simulink model "sim_sys_scara"  (R2017a)
settings: Solver=VariableStepAuto  StartTime=0.0  StopTime=4.1  MaxStep=0.01  RelTol=1e-4  EnableMultiTasking=on
values from neighbouring files (symbols this model uses):
  n_juncoes = size(vars, 1)    [animation.m]    (also in puma.m = 4; scara.m = 4)
undefined symbols (not defined in the file or in its folder): Q0
libraries: simulink x1
settings Model: Creator=julio  LastModifiedBy=julio
settings DataIOCC: LimitDataPoints=on  SaveOutput=off  SaveTime=off
settings OptimizationCC: ExpressionDepthLimit=2147483647  LifeSpan=1
settings DebuggingCC: AlgebraicLoopMsg=none  UnderspecifiedInitializationDetection=Classic  MergeDetectMultiDrivingBlocksExec=none  FcnCallInpInsideContextMsg=warning  AllowSymbolicDim=off  StateNameClashWarn=warning  SFUnexpectedBacktrackingDiag=warning  SFNoUnconditionalDefaultTransitionDiag=warning  SFExecutionAtInitializationDiag=none
settings GRTTargetCC: TargetLangStandard=C89/C90 (ANSI)  GeneratePreprocessorConditionals=Disable all  CombineOutputUpdateFcns=off  GRTInterface=on

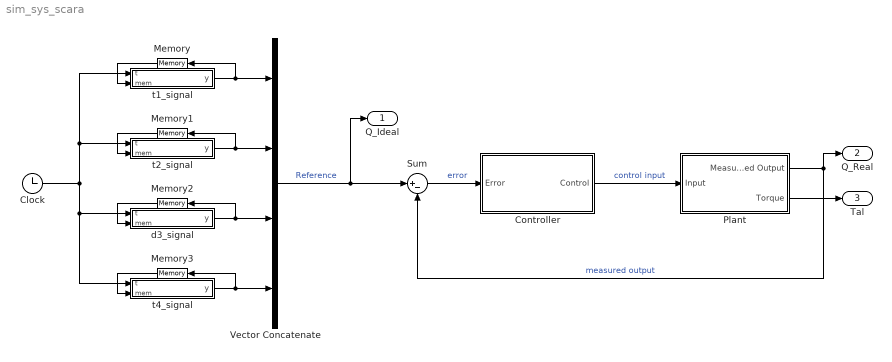
== system sim_sys_scara ==
  Clock : Clock
  Controller : Subsystem
  Memory : Memory  X0=Q0(1)
  Memory1 : Memory  X0=Q0(2)
  Memory2 : Memory  X0=Q0(3)
  Memory3 : Memory  X0=Q0(4)
  Plant : Subsystem
  Sum : Sum  Inputs=|+-
  Vector Concatenate : Concatenate  NumInputs=4
  d3_signal : MATLAB Function  TreatAsAtomicUnit=on
  t1_signal : MATLAB Function  TreatAsAtomicUnit=on
  t2_signal : MATLAB Function  TreatAsAtomicUnit=on
  t4_signal : MATLAB Function  TreatAsAtomicUnit=on
  Q_Ideal : Outport
  Q_Real : Outport  Port=2
  Tal : Outport  Port=3
  wires:
  Plant/1(Measured Output) -> Sum/2, Q_Real/1  "measured output"
  Sum/1 -> Controller/1(Error)  "error"
  Controller/1(Control) -> Plant/1(Input)  "control input"
  Vector Concatenate/1 -> Q_Ideal/1, Sum/1  "Reference"
  t1_signal/1(y) -> Memory/1, Vector Concatenate/1
  Memory/1 -> t1_signal/2(mem)
  Memory1/1 -> t2_signal/2(mem)
  t2_signal/1(y) -> Vector Concatenate/2, Memory1/1
  Memory2/1 -> d3_signal/2(mem)
  d3_signal/1(y) -> Vector Concatenate/3, Memory2/1
  Memory3/1 -> t4_signal/2(mem)
  t4_signal/1(y) -> Vector Concatenate/4, Memory3/1
  Clock/1 -> d3_signal/1(t), t4_signal/1(t), t2_signal/1(t), t1_signal/1(t)
  Plant/2(Torque) -> Tal/1

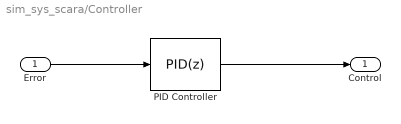
== system sim_sys_scara/Controller ==
  Error : Inport  PortDimensions=n_juncoes
  PID Controller : simulink/Continuous/PID Controller  Controller=PID  TimeDomain=Discrete-time  SampleTime=0.01  IntegratorMethod=Forward Euler  FilterMethod=Forward Euler  Form=Ideal  UseFilter=off  ControllerParametersSource=internal  P=8  I=5  D=10  N=20  InitialConditionSource=internal  InitialConditionForIntegrator=0  InitialConditionForFilter=0  ExternalReset=none  LimitOutput=off  UpperSaturationLimit=inf  LowerSaturationLimit=-inf  LinearizeAsGain=on  AntiWindupMode=none  Kb=1  TrackingMode=off  Kt=1  PParamMin=[]  PParamMax=[]  IParamMin=[]  IParamMax=[]  DParamMin=[]  DParamMax=[]  NParamMin=[]  NParamMax=[]  KbParamMin=[]  KbParamMax=[]  KtParamMin=[]  KtParamMax=[]  POutMin=[]  POutMax=[]  IOutMin=[]  IOutMax=[]  DOutMin=[]  DOutMax=[]  NOutMin=[]  NOutMax=[]  KbOutMin=[]  KbOutMax=[]  KtOutMin=[]  KtOutMax=[]  IntegratorOutMin=[]  IntegratorOutMax=[]  FilterOutMin=[]  FilterOutMax=[]  SumOutMin=[]  SumOutMax=[]  SumI1OutMin=[]  SumI1OutMax=[]  SumI2OutMin=[]  SumI2OutMax=[]  SumI3OutMin=[]  SumI3OutMax=[]  SumDOutMin=[]  SumDOutMax=[]  SaturationOutMin=[]  SaturationOutMax=[]  IntegratorContinuousStateAttributes=''  IntegratorStateMustResolveToSignalObject=off  IntegratorRTWStateStorageClass=Auto  FilterContinuousStateAttributes=''  FilterStateMustResolveToSignalObject=off  FilterRTWStateStorageClass=Auto  DifferentiatorICPrevScaledInput=0  DifferentiatorOutMin=[]  DifferentiatorOutMax=[]  InitialConditionSetting=State (most efficient)
  Control : Outport  PortDimensions=n_juncoes
  wires:
  Error/1 -> PID Controller/1
  PID Controller/1 -> Control/1

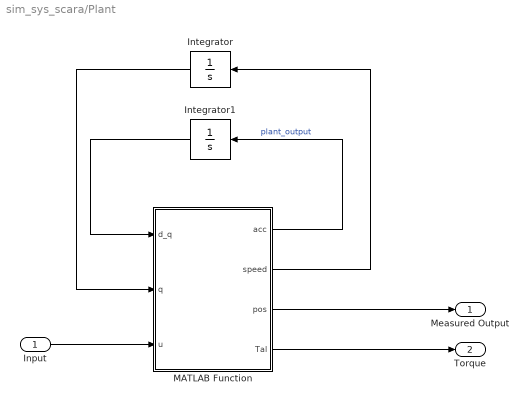
== system sim_sys_scara/Plant ==
  Input : Inport  PortDimensions=n_juncoes
  Integrator : Integrator  InitialCondition=Q0
  Integrator1 : Integrator  InitialCondition=zeros(n_juncoes, 1)
  MATLAB Function : MATLAB Function  TreatAsAtomicUnit=on
  Measured Output : Outport  PortDimensions=n_juncoes
  Torque : Outport  Port=2  PortDimensions=n_juncoes
  wires:
  Input/1 -> MATLAB Function/3(u)
  MATLAB Function/2(speed) -> Integrator/1
  MATLAB Function/1(acc) -> Integrator1/1  "plant_output"
  MATLAB Function/3(pos) -> Measured Output/1
  Integrator/1 -> MATLAB Function/2(q)
  Integrator1/1 -> MATLAB Function/1(d_q)
  MATLAB Function/4(Tal) -> Torque/1

== matlab function sim_sys_scara/t1_signal ==
  data: t input; y output; mem input
function y = fcn(t, mem)
    
    dt = 0.3;
    tempos = [
        [0,       1]
        [1+dt,   2.5+dt]
        [2.5+2*dt, 3.5+2*dt]
    ];

    period = max(max(tempos));
    t = mod(t,period);
    
    c = [
        [ -4727165597694197/144115188075855872,                               0,                                 0, -7549469994632933/9007199254740992,  1415525623993675/1125899906842624,   -283105124798735/562949953421312]
        [     -1028541733535679/70368744177664, 1491373747417675/35184372088832, -6719376224629081/140737488355328,     451928027705135/17592186044416, -7383929917174803/1125899906842624,   720383406553639/1125899906842624]
        [        1357713178735047/549755813888,  -1934191348076659/549755813888,      547843340131861/274877906944,    -2466787682990203/4398046511104,    5517226399439619/70368744177664, -4904201243946303/1125899906842624]

    ];

    i = 0;
    
    for j=1:size(tempos,1)
        if(t >= tempos(j,1))
            if t<= tempos(j,2)
                i = j;
                break;
            end
        end
    end
    
    if i> 0
        y = c(i,1) + c(i,2)*t + c(i,3)*t^2 + c(i,4)*t^3 + c(i,5)*t^4 + c(i,6)*t^5;
    else
        y = mem;
    end
    
end

== matlab function sim_sys_scara/Plant/MATLAB Function ==
  data: d_q input; acc output; q input; speed output; u input size=n_juncoes; pos output; Tal output
function [acc, speed, pos, Tal] = system(d_q, q, u)

    t1 = q(1);
    t2 = q(2);
    w1 = d_q(1);
    w2 = d_q(2);
    
    D = [
        [ (231*cos(t2))/80 + 6723/1600, (231*cos(t2))/160 + 903/800, 0, -1/100]
        [  (231*cos(t2))/160 + 903/800,                     903/800, 0, -1/100]
        [                            0,                           0, 8,      0]
        [                       -1/100,                      -1/100, 0,  1/100]
    ];

    C = [
        [ -(231*w2*sin(t2))/160, -(231*sin(t2)*(w1 + w2))/160, 0, 0]
        [  (231*w1*sin(t2))/160,                            0, 0, 0]
        [                     0,                            0, 0, 0]
        [                     0,                            0, 0, 0]
    ];

    g = [
                 0
                 0
          -78.4800
                 0
    ];
    acc = u;
    Tal = D*u + C*d_q + g;
    speed = d_q;
    pos = q;
end

== matlab function sim_sys_scara/t2_signal ==
  data: t input; y output; mem input
function y = fcn(t,mem)
    
    dt = 0.3;
    tempos = [
        [0,       1]
        [1+dt,   2.5+dt]
        [2.5+2*dt, 3.5+2*dt]
    ];

    period = max(max(tempos));
    t = mod(t,period);
    
    c = [
        [ 5162075642626993/2251799813685248,                                               0,                                                0,                 -765116889043487/70368744177664,                  4590701334260921/281474976710656,                 -3672561067408737/562949953421312]
        [ 5427403195375643/4503599627370496, 3683388495235123/316912650057057350374175801344, -4148871656720877/316912650057057350374175801344, 2232339815295405/316912650057057350374175801344, -2279599811385095/1267650600228229401496703205376, 7116799411153465/40564819207303340847894502572032]
        [    -2032241429182977/549755813888,                      90527431081067/17179869184,                   -1641032267590695/549755813888,                  3694558177989231/4398046511104,                  -2065815600428863/17592186044416,                  3672561067429071/562949953421312]
    ];

    i = 0;
    
    for j=1:size(tempos,1)
        if(t >= tempos(j,1))
            if t<= tempos(j,2)
                i = j;
                break;
            end
        end
    end
    
    if i> 0
        y = c(i,1) + c(i,2)*t + c(i,3)*t^2 + c(i,4)*t^3 + c(i,5)*t^4 + c(i,6)*t^5;
    else
        y = mem;
    end
    
end

== matlab function sim_sys_scara/d3_signal ==
  data: t input; y output; mem input
function y = fcn(t,mem)
    
    dt = 0.3;
    tempos = [
        [0,       1]
        [1+dt,   2.5+dt]
        [2.5+2*dt, 3.5+2*dt]
    ];

    period = max(max(tempos));
    t = mod(t,period);
    
    c = [
        [1.2000         0         0         0         0         0]
        [1.2000         0         0         0         0         0]
        [1.2000         0         0         0         0         0]
    ];

    i = 0;
    
    for j=1:size(tempos,1)
        if(t >= tempos(j,1))
            if t<= tempos(j,2)
                i = j;
                break;
            end
        end
    end
    
    if i> 0
        y = c(i,1) + c(i,2)*t + c(i,3)*t^2 + c(i,4)*t^3 + c(i,5)*t^4 + c(i,6)*t^5;
    else
        y = mem;
    end
    
end

== matlab function sim_sys_scara/t4_signal ==
  data: t input; y output; mem input
function y = fcn(t,mem)
    
    dt = 0.3;
    tempos = [
        [0,       1]
        [1+dt,   2.5+dt]
        [2.5+2*dt, 3.5+2*dt]
    ];

    period = max(max(tempos));
    t = mod(t,period);
    
    c = [
        [1     0     0     0     0     0]
        [1     0     0     0     0     0]
        [1     0     0     0     0     0]
    ];

    i = 0;
    
    for j=1:size(tempos,1)
        if(t >= tempos(j,1))
            if t<= tempos(j,2)
                i = j;
                break;
            end
        end
    end
    
    if i> 0
        y = c(i,1) + c(i,2)*t + c(i,3)*t^2 + c(i,4)*t^3 + c(i,5)*t^4 + c(i,6)*t^5;
    else
        y = mem;
    end
    
end
